simulink subsystem "Forces_and_Moments"  (R2024b)
settings: Solver=VariableStepAuto  StartTime=0.0  StopTime=10.0  RelTol=1e-3
undefined symbols (not defined in the file or in its folder): canard_pos_r_mean, rocket_diameter
settings Model: Creator=joedo  LastModifiedBy=finnb

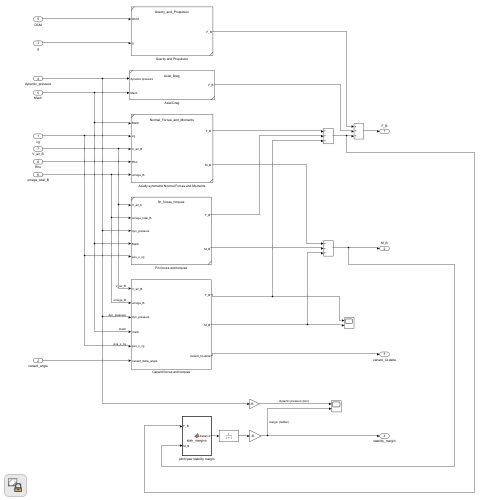
[thumbnail: Simulink's stored preview of the top-level diagram]
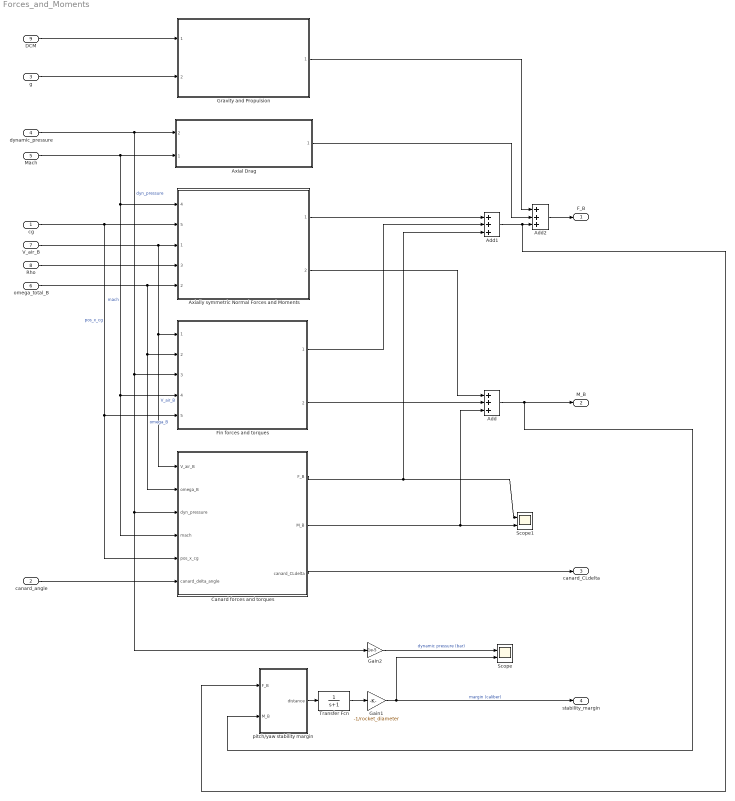
== system Forces_and_Moments ==
  cg : Inport
  canard_angle : Inport  Port=2
  g : Inport  Port=3
  "dynamic_pressure " : Inport  Port=4
  Mach : Inport  Port=5
  omega_total_B : Inport  Port=6
  V_air_B : Inport  Port=7
  Rho : Inport  Port=8
  DCM : Inport  Port=9
  Add : Sum  Inputs=+++
  Add1 : Sum  Inputs=+++
  Add2 : Sum  Inputs=+++
  Axial Drag : Subsystem  ReferencedSubsystem=Axial_Drag
      settings: PortSchema="{\"entries\":[{\"content\":{\"sides\":[{\"content\":{\"connectorIds\":[\"In2\",\"In1\"]},\"type\":\"ConnectorPlacement.EquallySpacedRectSide\",\"uuid\":\"98f34f10-6b70-49d4-9473-053176858c1a\"},{\"content\":{\"connectorIds\":[\"Out1\"],\"side\":\"RIGHT\"},\"type\":\"ConnectorPlacement.EquallySpacedRectSide\",\"uuid\":\"814cea4a-822c-4810-b2b2-e02e175f38ce\"},{\"content\":{\"side\":\"TOP\"},\"type\":\"ConnectorPlacement.EquallySpacedRectSide\",\"uuid\":\"80808368-ed63-4ba9-a98f-5e59c93983e4\"}]},\"type\":\"ConnectorPlacement.EquallySpacedConnector\",\"uuid\":\"073858c7-1f90-4321-8d7b-b9f324961e15\"}],\"packageUris\":[\"http://schema.mathworks.com/mf0/Connector/R2020b\"],\"version\":\"1.0\"}"
  Axially symmetric Normal Forces and Moments : Subsystem  ReferencedSubsystem=Normal_Forces_and_Moments
      settings: PortSchema="{\"entries\":[{\"content\":{\"sides\":[{\"content\":{\"connectorIds\":[\"In4\",\"In5\",\"In1\",\"In3\",\"In2\"]},\"type\":\"ConnectorPlacement.EquallySpacedRectSide\",\"uuid\":\"3d060e6d-6cf3-4341-877b-3cb591774c08\"},{\"content\":{\"connectorIds\":[\"Out1\",\"Out2\"],\"side\":\"RIGHT\"},\"type\":\"ConnectorPlacement.EquallySpacedRectSide\",\"uuid\":\"12a83e93-0b1c-4946-a0d1-6eef9ce0d7d5\"},{\"content\":{\"side\":\"TOP\"},\"type\":\"ConnectorPlacement.EquallySpacedRectSide\",\"uuid\":\"237cf4f0-7c1b-4235-9d1e-c459b6944e6b\"}]},\"type\":\"ConnectorPlacement.EquallySpacedConnector\",\"uuid\":\"ee604e45-0548-4bf4-9ee4-77069ab5adfd\"}],\"packageUris\":[\"http://schema.mathworks.com/mf0/Connector/R2020b\"],\"version\":\"1.0\"}"
  Canard forces and torques : Subsystem
  Fin forces and torques : Subsystem  ReferencedSubsystem=fin_forces_torques
  Gain1 : Gain  Gain=-1/rocket_diameter
  Gain2 : Gain  Gain=1e-5
  Gravity and Propulsion : Subsystem  ReferencedSubsystem=Gravity_and_Propulsion
  Scope : Scope  NumInputPorts=2
  Scope1 : Scope  NumInputPorts=2
  Transfer Fcn : TransferFcn  Denominator=[1 1]
  pitch/yaw stability margin : MATLAB Function  TreatAsAtomicUnit=on
  F_B : Outport  VectorParamsAs1DForOutWhenUnconnected=off
  M_B : Outport  Port=2  VectorParamsAs1DForOutWhenUnconnected=off
  canard_CLdelta : Outport  Port=3
  stability_margin : Outport  Port=4
  wires:
  V_air_B/1 -> Axially symmetric Normal Forces and Moments/1, Canard forces and torques/1(V_air_B), Fin forces and torques/1  "V_air_B"
  Mach/1 -> Canard forces and torques/4(mach), Fin forces and torques/4, Axially symmetric Normal Forces and Moments/4, Axial Drag/1  "mach"
  omega_total_B/1 -> Canard forces and torques/2(omega_B), Fin forces and torques/2, Axially symmetric Normal Forces and Moments/2  "omega_B"
  "dynamic_pressure "/1 -> Axial Drag/2, Fin forces and torques/3, Canard forces and torques/3(dyn_pressure), Gain2/1  "dyn_pressure"
  Rho/1 -> Axially symmetric Normal Forces and Moments/3
  Gravity and Propulsion/1 -> Add2/1
  DCM/1 -> Gravity and Propulsion/1
  Axial Drag/1 -> Add2/2
  Axially symmetric Normal Forces and Moments/1 -> Add1/1
  Axially symmetric Normal Forces and Moments/2 -> Add/1
  g/1 -> Gravity and Propulsion/2
  cg/1 -> Canard forces and torques/5(pos_x_cg), Fin forces and torques/5, Axially symmetric Normal Forces and Moments/5  "pos_x_cg"
  Fin forces and torques/1 -> Add1/2
  Fin forces and torques/2 -> Add/2
  canard_angle/1 -> Canard forces and torques/6(canard_delta_angle)
  Canard forces and torques/2(M_B) -> Scope1/2, Add/3
  Canard forces and torques/3(canard_CLdelta) -> canard_CLdelta/1
  Canard forces and torques/1(F_B) -> Scope1/1, Add1/3
  pitch/yaw stability margin/1(distance) -> Transfer Fcn/1
  Add2/1 -> F_B/1
  Add1/1 -> Add2/3, pitch/yaw stability margin/1(F_B)
  Add/1 -> pitch/yaw stability margin/2(M_B), M_B/1
  Transfer Fcn/1 -> Gain1/1
  Gain1/1 -> Scope/2, stability_margin/1  "margin (caliber)"
  Gain2/1 -> Scope/1  "dynamic pressure (bar)"

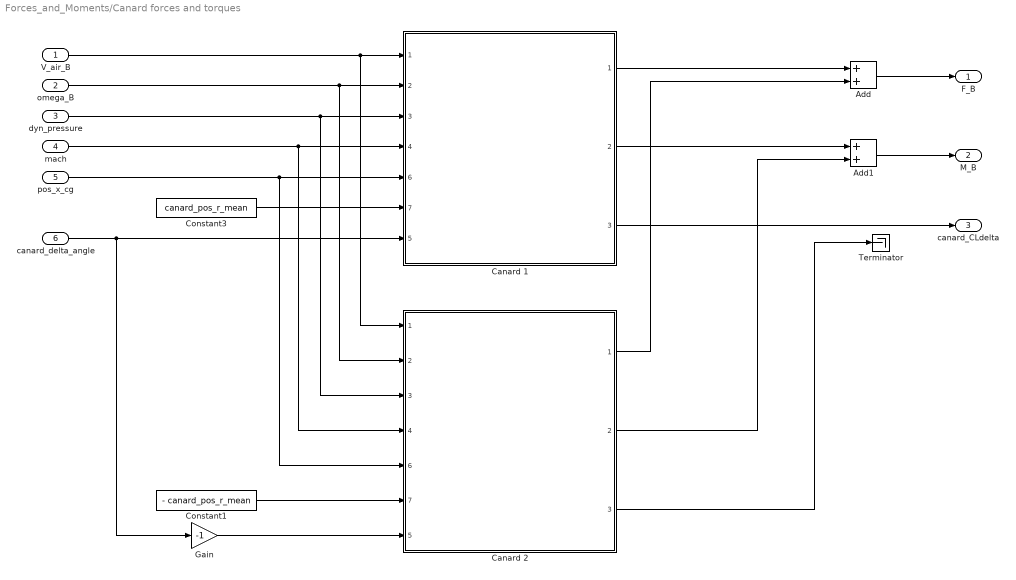
== system Forces_and_Moments/Canard forces and torques ==
  V_air_B : Inport
  omega_B : Inport  Port=2
  dyn_pressure : Inport  Port=3
  mach : Inport  Port=4
  pos_x_cg : Inport  Port=5
  canard_delta_angle : Inport  Port=6
  Add : Sum
  Add1 : Sum
  Canard 1 : Subsystem  ReferencedSubsystem=canard_forces_torques
      settings: PortSchema="{\"entries\":[{\"content\":{\"sides\":[{\"content\":{\"connectorIds\":[\"In1\",\"In2\",\"In3\",\"In4\",\"In6\",\"In7\",\"In5\"]},\"type\":\"ConnectorPlacement.EquallySpacedRectSide\",\"uuid\":\"fbe3b5f2-d9a4-4468-a335-6367ffdd4d60\"},{\"content\":{\"connectorIds\":[\"Out1\",\"Out2\",\"Out3\"],\"side\":\"RIGHT\"},\"type\":\"ConnectorPlacement.EquallySpacedRectSide\",\"uuid\":\"de5d3007-d105-406a-89bb-cc0c7eab64f0\"},{\"content\":{\"side\":\"TOP\"},\"type\":\"ConnectorPlacement.EquallySpacedRectSide\",\"uuid\":\"df0e13ca-9df7-4bc2-b76b-3c11bd5b2d07\"}]},\"type\":\"ConnectorPlacement.EquallySpacedConnector\",\"uuid\":\"d33a9aea-379e-46de-adf5-e874e082a497\"}],\"packageUris\":[\"http://schema.mathworks.com/mf0/Connector/R2020b\"],\"version\":\"1.0\"}"
  Canard 2 : Subsystem  ReferencedSubsystem=canard_forces_torques
      settings: PortSchema="{\"entries\":[{\"content\":{\"sides\":[{\"content\":{\"connectorIds\":[\"In1\",\"In2\",\"In3\",\"In4\",\"In6\",\"In7\",\"In5\"]},\"type\":\"ConnectorPlacement.EquallySpacedRectSide\",\"uuid\":\"fbe3b5f2-d9a4-4468-a335-6367ffdd4d60\"},{\"content\":{\"connectorIds\":[\"Out1\",\"Out2\",\"Out3\"],\"side\":\"RIGHT\"},\"type\":\"ConnectorPlacement.EquallySpacedRectSide\",\"uuid\":\"de5d3007-d105-406a-89bb-cc0c7eab64f0\"},{\"content\":{\"side\":\"TOP\"},\"type\":\"ConnectorPlacement.EquallySpacedRectSide\",\"uuid\":\"df0e13ca-9df7-4bc2-b76b-3c11bd5b2d07\"}]},\"type\":\"ConnectorPlacement.EquallySpacedConnector\",\"uuid\":\"d33a9aea-379e-46de-adf5-e874e082a497\"}],\"packageUris\":[\"http://schema.mathworks.com/mf0/Connector/R2020b\"],\"version\":\"1.0\"}"
  Constant1 : Constant  Value=- canard_pos_r_mean
  Constant3 : Constant  Value=canard_pos_r_mean
  Gain : Gain  Gain=-1
  Terminator : Terminator
  F_B : Outport
  M_B : Outport  Port=2
  canard_CLdelta : Outport  Port=3
  wires:
  pos_x_cg/1 -> Canard 2/6, Canard 1/6
  Add1/1 -> M_B/1
  Add/1 -> F_B/1
  Canard 1/3 -> canard_CLdelta/1
  Canard 2/3 -> Terminator/1
  Gain/1 -> Canard 2/5
  Canard 2/2 -> Add1/2
  Canard 1/1 -> Add/1
  canard_delta_angle/1 -> Canard 1/5, Gain/1
  omega_B/1 -> Canard 1/2, Canard 2/2
  V_air_B/1 -> Canard 1/1, Canard 2/1
  Canard 2/1 -> Add/2
  mach/1 -> Canard 1/4, Canard 2/4
  Canard 1/2 -> Add1/1
  Constant1/1 -> Canard 2/7
  Constant3/1 -> Canard 1/7
  dyn_pressure/1 -> Canard 1/3, Canard 2/3

== matlab function Forces_and_Moments/pitch//yaw stability margin ==
  data: F_B input; M_B input; distance output
function distance  = stab_margins(F_B, M_B)
    
    % only absolute normal force, torque
    
    % project to x-normal plane
    F_yz = F_B(2:3);
    M_yz = M_B(2:3);

    % find magnitude and normal direction of net forces, moment
    F_mag = norm(F_yz);
    F_dir = atan2(F_yz(1), F_yz(2));
    M_mag = norm(M_yz);
    M_dir = atan2(M_yz(1), M_yz(2));
    
    % find main axes of force
    R = @(angle) [cos(angle), -sin(angle); sin(angle), cos(angle)];
    F_main = R(F_dir) * F_yz;
    M_main = R(F_dir) * M_yz;

    F = F_main(2);
    M = M_main(1);

    % exclude no force
    if F ~= 0
        distance = M / F;
    else 
        distance = -10; % arbitrary large value for no normal force
    end

end

% Body relative velocity magnitude
    % Vrel_mag = norm(Vrel);
    % Vrel_X = Vrel(1);
    % Vrel_magYZ = norm(Vrel(2:3));
    % 
    % incidence = atan2(Vrel_magYZ, Vrel_X);
